simulink model "sistema"  (R2026a)
settings: Solver=VariableStepAuto
settings Model: Creator=BioMath  LastModifiedBy=BioMath
settings DataIOCC: TimeSaveName=t
settings DebuggingCC: ArtificialAlgebraicLoopMsg=none  MaxConsecutiveZCsMsg=none

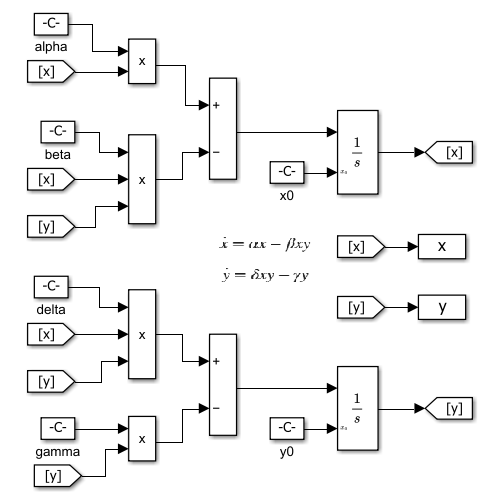
[thumbnail: Simulink's stored preview of the top-level diagram]
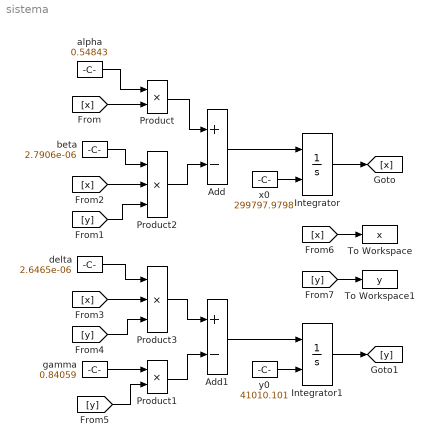
== system sistema ==
  Add : Sum  Inputs=+-
  Add1 : Sum  Inputs=+-
  Integrator : Integrator  InitialConditionSource=external
  Integrator1 : Integrator  InitialConditionSource=external
  Product : Product
  Product1 : Product
  Product2 : Product  Inputs=3
  Product3 : Product  Inputs=3
  To Workspace : ToWorkspace  VariableName=x  SampleTime=-1
  To Workspace1 : ToWorkspace  VariableName=y  SampleTime=-1
  alpha : Constant  Value=0.54843
  beta : Constant  Value=2.7906e-06
  delta : Constant  Value=2.6465e-06
  gamma : Constant  Value=0.84059
  x0 : Constant  Value=299797.9798
  y0 : Constant  Value=41010.101
  wires:
  Add1/1 -> Integrator1/1
  Add/1 -> Integrator/1
  x0/1 -> Integrator/2
  y0/1 -> Integrator1/2
  Integrator/1 -> [x]
  Integrator1/1 -> [y]
  Product2/1 -> Add/2
  Product/1 -> Add/1
  Product3/1 -> Add1/1
  Product1/1 -> Add1/2
  [x] -> Product/2
  alpha/1 -> Product/1
  [x] -> Product2/2
  beta/1 -> Product2/1
  [y] -> Product2/3
  [x] -> Product3/2
  [y] -> Product3/3
  delta/1 -> Product3/1
  gamma/1 -> Product1/1
  [y] -> Product1/2
  [x] -> To Workspace/1
  [y] -> To Workspace1/1
